simulink model "load_arduino_v_15_loop"  (R2020b)
settings: Solver=FixedStepDiscrete  StartTime=0.0  StopTime=Inf  FixedStep=0.02  RelTol=1e-3  EnableMultiTasking=on
values from neighbouring files (symbols this model uses):
  attuatore_Amax = deg2rad(20)    [AVVIO_YAK_DATA.m]
  attuatore_Amin = deg2rad(-20)    [AVVIO_YAK_DATA.m]
  attuatore_Emax = deg2rad(25)    [AVVIO_YAK_DATA.m]
  attuatore_Emin = deg2rad(-25)    [AVVIO_YAK_DATA.m]
  attuatore_Rmax = deg2rad(25)    [AVVIO_YAK_DATA.m]
  attuatore_Rmin = deg2rad(-25)    [AVVIO_YAK_DATA.m]
  attuatore_Tmax = 0.4    [AVVIO_YAK_DATA.m]
  attuatore_Tmin = 0    [AVVIO_YAK_DATA.m]
  interventoA_05 = 6    [AVVIO_YAK_DATA.m]
  interventoA_1 = 2    [AVVIO_YAK_DATA.m]
  interventoE_05 = 7.5    [AVVIO_YAK_DATA.m]
  interventoE_1 = 3.2    [AVVIO_YAK_DATA.m]
  interventoT = 0.1    [AVVIO_YAK_DATA.m]
  inv_A = 1    [AVVIO_YAK_DATA.m]
  inv_comp_h = 1    [AVVIO_YAK_DATA.m]
  inv_E = 1    [AVVIO_YAK_DATA.m]
  inv_R = 1    [AVVIO_YAK_DATA.m]
  inv_T = 1    [AVVIO_YAK_DATA.m]
  K_AW_B_AP_quota = 1000    [AVVIO_YAK_DATA.m]
  K_AW_B_becc = -250    [AVVIO_YAK_DATA.m]
  K_AW_B_imb = 0    [AVVIO_YAK_DATA.m]
  K_AW_B_roll = 500    [AVVIO_YAK_DATA.m]
  K_imb_inv = -1    [AVVIO_YAK_DATA.m]
  Kd_h_app = 0.085    [AVVIO_YAK_DATA.m]
  Kd_h_flare = 0.01    [AVVIO_YAK_DATA.m]
  Ki_AP_quota_select = 0.014    [AVVIO_YAK_DATA.m]
  Ki_AP_rotta = 0.03    [AVVIO_YAK_DATA.m]
  Ki_AP_vel = 0.001    [AVVIO_YAK_DATA.m]
  Ki_becch = -0.064065    [AVVIO_YAK_DATA.m]
  Ki_h_app = 0.055    [AVVIO_YAK_DATA.m]
  Ki_h_cruise = 0.008    [AVVIO_YAK_DATA.m]
  Ki_h_flare = 0.07    [AVVIO_YAK_DATA.m]
  Ki_roll = 0.025    [AVVIO_YAK_DATA.m]
  Kp_AP_quota_hold_h = 0.15    [AVVIO_YAK_DATA.m]
  Kp_AP_quota_hold_l = 0.7    [AVVIO_YAK_DATA.m]
  Kp_AP_quota_select = 0.014    [AVVIO_YAK_DATA.m]
  Kp_AP_rotta = 0.7    [AVVIO_YAK_DATA.m]
  Kp_AP_vel = 0.02692    [AVVIO_YAK_DATA.m]
  Kp_becch = -0.1918    [AVVIO_YAK_DATA.m]
  Kp_comp_h = 0.035    [AVVIO_YAK_DATA.m]
  Kp_h_app_max = 0.086    [AVVIO_YAK_DATA.m]
  Kp_h_app_min = 0.01    [AVVIO_YAK_DATA.m]
  Kp_h_cruise = 0.04    [AVVIO_YAK_DATA.m]
  Kp_h_flare = 0.1    [AVVIO_YAK_DATA.m]
  Kp_imb = -0.04    [AVVIO_YAK_DATA.m]
  Kp_p = 0.025    [AVVIO_YAK_DATA.m]
  Kp_q = -0.025    [AVVIO_YAK_DATA.m]
  Kp_roll = 0.11    [AVVIO_YAK_DATA.m]
  Kp_Rotta_ATO = 4    [AVVIO_YAK_DATA.m]
  safe_phi = 55    [AVVIO_YAK_DATA.m]
  safe_V = 40    [AVVIO_YAK_DATA.m]
  t_AP = 0.02    [AVVIO_YAK_DATA.m]
  time_alarm_SAFE = 1    [AVVIO_YAK_DATA.m]
  V_max = 35    [AVVIO_YAK_DATA.m]
  V_stall = 15    [AVVIO_YAK_DATA.m]
  vel_wp1_al = 25    [AVVIO_YAK_DATA.m]
  vel_wp2_al = 20    [AVVIO_YAK_DATA.m]
undefined symbols (not defined in the file or in its folder): DiscIntNeverNeededParam, Newton, phi_max, phi_min, Raphson, theta_max, theta_min, tsamp
libraries: simulink_extras x43, arduinolib x26, pid_lib x8, svdutilitieslib x6, simulink x3, dspsigops x3, aerolibtransform2sys x2, aerolibtransform2 x2, cstblocks x1
(part 6 of 8)

== matlab function load_arduino_v_15_loop/AUTOPILOTA/Subsystem1/Subsystem1/APPROACH/MATLAB Function ==
  data: reset input; gamma input; x_f_out output; h_f_out output; xg0 input; k_x_out output; h_c_out output; no_solution output
function [x_f_out,h_f_out,k_x_out,h_c_out,no_solution] = fcn(reset,gamma,xg0)

 

x_f=-200;
h_f=1.5;
%x_f=-300;
%h_f=10;
k_x=0.01;
h_c=-2;
x_td=5;
h_td_dot=-0.1;
x_td_dot=18;
no_solution = 0;

% x_f=-200;
% h_f=5;
% %x_f=-300;
% %h_f=10;
% k_x=0.01;
% h_c=-1;
% x_td=50;
% h_td_dot=-0.15;
% x_td_dot=18;
% no_solution = 0;

% F = [f(x_f,h_f,gamma,xg0); g(h_c,h_f,k_x,gamma); r(h_c,h_f,k_x,x_f,x_td); s(h_c,h_f,k_x,x_f,x_td,h_td_dot,x_td_dot)];
% 
% J = [ df1() df2(gamma) df3() df4();
%       dg1(k_x) dg2() dg3(h_f,h_c) dg4(k_x);
%       dr1(k_x,x_td,x_f) dr2(k_x,x_td,x_f) dr3(k_x,x_td,x_f,h_f,h_c) dr4();
%       ds1(k_x,x_td,x_f,x_td_dot) ds2(k_x,x_td,x_f,x_td_dot,h_f,h_c) ds3(k_x,x_td,x_f,x_td_dot,h_f,h_c) ds4(k_x,x_td,x_f,x_td_dot)]

persistent x x_new cycle_count eps

if (isempty(x) ||  reset == 0)
x = [h_f; x_f; k_x; h_c];
end

if (isempty(x_new) || reset == 0)
x_new = zeros(4,1);
end

if (isempty(eps) || reset == 0)
eps = ones(1,4);
end
   
if (isempty(cycle_count) || reset == 0)
cycle_count = 0;
end




while ~ (eps(1) < 0.1 && eps(2) < 0.1 && eps(3) < 0.1 && eps(4) < 0.1 )

F = [f(x(2),x(1),gamma,xg0); g(x(4),x(1),x(3),gamma); r(x(4),x(1),x(3),x(2),x_td); s(x(4),x(1),x(3),x(2),x_td,h_td_dot,x_td_dot)];

J = [ df1() df2(gamma) df3() df4();
      dg1(x(3)) dg2() dg3(x(1),x(4)) dg4(x(3));
      dr1(x(3),x_td,x(2)) dr2(x(3),x_td,x(2),x(1),x(4)) dr3(x(3),x_td,x(2),x(1),x(4)) dr4();
      ds1(x(3),x_td,x(2),x_td_dot) ds2(x(3),x_td,x(2),x_td_dot,x(1),x(4)) ds3(x(3),x_td,x(2),x_td_dot,x(1),x(4)) ds4(x(3),x_td,x(2),x_td_dot)] ; 
  
  
x_new = x - J^(-1)*F;

eps(1) = abs(x_new(1)-x(1));
eps(2) = abs(x_new(2)-x(2));
eps(3) = abs(x_new(3)-x(3));
eps(4) = abs(x_new(4)-x(4));


x = x_new;

cycle_count = cycle_count + 1;

if cycle_count > 10
   no_solution = 1; 
   break; 
end

end

if (eps(1) < 0.1 && eps(2) < 0.1 && eps(3) < 0.1 && eps(4) < 0.1 )
   
h_f_out = x(1);
x_f_out = x(2);
k_x_out = x(3);
h_c_out = x(4);

else
    
h_f_out = 0;
x_f_out = 0;
k_x_out = 0;
h_c_out = 0;    
end

function y = f(x_f,h_f,gamma,xg0)                 %inizio equazioni sistema non lineare
y = h_f+(x_f-xg0)*tan(gamma);
end

function y = g(h_c,h_f,k_x,gamma)
y = (h_f-h_c)*k_x-tan(gamma);
end

function y = r(h_c,h_f,k_x,x_f,x_td)
y = h_c + (h_f-h_c)*exp(-k_x*(x_td-x_f));
end

function y = s(h_c,h_f,k_x,x_f,x_td,h_td_dot,x_td_dot)
y = h_td_dot + (h_f-h_c)*k_x*x_td_dot*exp(-k_x*(x_td-x_f));        
end                                                                   % fine equazioni sistema non lineare

function y = df1()                                                    %inizio derivate
y = 1;
end

function y = df2(gamma)
y = tan(gamma);
end

function y = df3()
y = 0;
end

function y = df4()
y = 0;
end

function y = dg1(k_x)
y = k_x;
end

function y = dg2()
y = 0;
end

function y = dg3(h_f,h_c)
y = h_f-h_c;
end

function y = dg4(k_x)
y = -k_x;
end

function y = dr1(k_x,x_td,x_f)
y = exp(-k_x*(x_td-x_f));
end

function y = dr2(k_x,x_td,x_f,h_f,h_c)
y = (h_f-h_c)*k_x*exp(-k_x*(x_td-x_f));
end

function y = dr3(k_x,x_td,x_f,h_f,h_c)
y = (h_f-h_c)*(x_f-x_td)*exp(-k_x*(x_td-x_f));
end

function y = dr4()
y = 1;
end

function y = ds1(k_x,x_td,x_f,x_td_dot)
y = k_x*x_td_dot*exp(-k_x*(x_td-x_f));
end

function y = ds2(k_x,x_td,x_f,x_td_dot,h_f,h_c)
y = (h_f-h_c)*k_x^2*x_td_dot*exp(-k_x*(x_td-x_f));
end

function y = ds3(k_x,x_td,x_f,x_td_dot,h_f,h_c)
y = (h_f-h_c)*x_td_dot*exp(-k_x*(x_td-x_f))+(h_f-h_c)*k_x*x_td_dot*(x_f-x_td)*exp(-k_x*(x_td-x_f));
end

function y = ds4(k_x,x_td,x_f,x_td_dot)
y = -k_x*x_td_dot*exp(-k_x*(x_td-x_f));
end



end

== matlab function load_arduino_v_15_loop/Misure Sensori/BMP_280/MATLAB Function ==
  data: rate_l_up output; Cal_alt input; P input; P_int input; P_refer output; P_cal input; rate_l_dw output
function [rate_l_up, P_refer, rate_l_dw]  = fcn( Cal_alt, P,P_int,P_cal)
%#codegen

persistent P_ref rl_up rl_dw

if isempty(P_ref)
    
    P_ref = 101325;
    
end

if isempty(rl_up)
    
    rl_up = 300;
    
end

if isempty(rl_dw)
    
    rl_dw = -300;
    
end

if Cal_alt == 1
    
    P_ref = P;
 
end

if P_int == 1
   
   P_ref = P_cal; 
   rl_up = 20;
   rl_dw = -20;
    
end
    


P_refer = P_ref;

rate_l_up = rl_up;
rate_l_dw = rl_dw;

== matlab function load_arduino_v_15_loop/Misure Sensori/GPS_Venus/Subsystem2/Create_message ==
  data: status output; byte_pack input; messaggio output
function [status,messaggio]  = LETTURA_NMEA(byte_pack)

persistent message counter start_found end_found

status = false;       %ho aggiunto questo
messaggio = uint8(zeros(1,80)) ;
pos_end = uint8(0) ;
M = uint8(length(byte_pack)) ;


if isempty(end_found) 
    end_found = false ;
end 
if isempty(start_found) 
     start_found = false ;
end 
if isempty (counter) 
    counter = uint8(0) ;
end 
if isempty(message)
     message = uint8(zeros(1,80)) ;
end



if start_found == 0 
    for i = uint8(1) : M  
        if byte_pack(i) == '$' 
            message(1:M - (i-1)) = byte_pack(i:end) ;
            counter = M - (i-1) ; 
            start_found = true ;
            break
        end
    end
    
    
elseif start_found == 1
    for i = uint8(1) : M  
        if byte_pack(i) == 13 
            end_found = true ;
            pos_end = i ;
            break
        end
    end
    
    if end_found == 1
        message(counter + 1 : counter + pos_end) = byte_pack(1:pos_end) ;
        status = true;       %ho aggiunto questo
        messaggio = message ;
        end_found = false ;
        counter = M - pos_end ;
        if pos_end == M 
            start_found = false ; 
            message = uint8(zeros(1,80)) ;
        else  
            start_found = true ;
            message(1:(M - pos_end)) = byte_pack(pos_end + 1 : end) ;
            message(M - pos_end +1 : 80) = ...
                uint8(zeros(1,80 - (M - pos_end) )) ;
        end
         

    else 
    message(counter + 1 : M + counter ) = byte_pack ;
    counter = M + counter  ;
   
    end
    
    
 
        
    
    
end

== matlab function load_arduino_v_15_loop/Misure Sensori/GPS_Venus/Subsystem2/Subsystem/MATLAB Function ==
  data: messaggio input; Lat output; Long output; V output; Magnetic_declination output; heading output; fix_mode output; n_sat output; h_mean_sea output; h_WGS84 output; out_prec input; indice_dimario output
function [Lat,Long,V,Magnetic_declination,heading,fix_mode,n_sat,h_mean_sea,h_WGS84,indice_dimario] = parser_NMEA(messaggio,out_prec)
    

messaggio = char(messaggio) ;

comma_gga = uint8(zeros(1,14));
comma_rmc = uint8(zeros(1,12));
star = uint8(0);
dollar = uint8(0);
find_dollar = uint8(0);
find_comma = uint8(0);
message_type = uint8(zeros(1,5));
indice_dimario = uint8(0);





for i=1:length(messaggio)
   if messaggio(i) == '$'
       find_dollar = find_dollar + uint8(1);
   end
   if messaggio(i) == ','
       find_comma = find_comma + uint8(1);
   end
end
    
if (find_dollar == 1 && (find_comma == 12 || find_comma == 14))               % controllo se il numero di $ e , sono corretti all'interno di messaggio
                                                                             % altrimenti il messaggio è corrotto ed in output mando i messaggi
                                                                             % precedenti
dollar= find(messaggio == '$',1);

mess_type = messaggio(dollar(1) + 1 : dollar(1) + 5);                              % è il nome del messaggio arrivato

% decodifica mesaggio RMC

if mess_type == 'GPRMC'
comma_rmc = find(messaggio == ',');                                              % restituisce le posizioni delle virgole all'interno del messaggio
star = find(messaggio == '*');                                               % restituisce la posizione dell'asterisco all'interno del messaggio
dollar = find(messaggio == '$');                                             % restituisce la posizione del dollaro all'interno del messaggio

Lat_1 = str2double(messaggio(comma_rmc(3) + 1 : comma_rmc(3) + 2));
Lat_2 = str2double(messaggio(comma_rmc(3) + 3 : comma_rmc(4) - 1))/60;
Lat = Lat_1 + Lat_2;
if messaggio(comma_rmc(4) + 1) == 'S'
Lat = -Lat; 
end

Long_1 = str2double(messaggio(comma_rmc(5) + 1 : comma_rmc(5) + 3));
Long_2 = str2double(messaggio(comma_rmc(5) + 4 : comma_rmc(6) - 1))/60;
Long = Long_1 + Long_2;
if messaggio(comma_rmc(6) + 1) == 'W'
Long = -Long; 
end

V = str2double(messaggio(comma_rmc(7) + 1 : comma_rmc(8) - 1)); 
    
heading = str2double(messaggio(comma_rmc(8) + 1 : comma_rmc(9) - 1));

Magnetic_declination = str2double(messaggio(comma_rmc(10) + 1 : comma_rmc(11) - 1));
if messaggio(comma_rmc(11) + 1) == 'W'
Magnetic_declination = -Magnetic_declination; 
end

% questi dati non sono presenti nel messaggio rmc, quindi prendo quelli
% precedenti

fix_mode = complex(out_prec(6),0);

n_sat = complex(out_prec(7),0) ;

h_mean_sea = complex(out_prec(8),0) ;

h_WGS84 = complex(out_prec(9),0) ;


%%%%%%%%%%%%%%%%%%%%%%%%%%%%%%%%%%%%%%%%%%%%%%%%%%%%%%%%%

% calcolo checksum

ck_ric = char(zeros(1,2)) ;
ck_ric(1) = messaggio(star(1) + uint8(1))  ;
ck_ric(2) = messaggio(star(1) + uint8(2)) ;

NMEA_rmc_string = uint8(messaggio(dollar(1)+1:star(1)-1)) ;

checksum = uint8(0) ;
for i = 1:length(NMEA_rmc_string) 
    checksum = bitxor(checksum,NMEA_rmc_string(i),'uint8') ;
end

if checksum ~= hex2dec(ck_ric) 
    Lat = out_prec(1) ;
    Long = out_prec(2) ;
    V = out_prec(3) ;
    Magnetic_declination = out_prec(4);
    heading = out_prec(5) ; 
    fix_mode = complex(out_prec(6),0);
    n_sat = complex(out_prec(7),0) ;
    h_mean_sea = complex(out_prec(8),0) ;
    h_WGS84 = complex(out_prec(9),0) ;
    indice_dimario = uint8(10);
end

%%%%%%%%%%%%%%%%%%%%%%%%%%%%%%%%%%%%%%%%%%%%%%%%%%%%%%%%%%%

% decodifica mesaggio GGA

elseif mess_type == 'GPGGA'
comma_gga = find(messaggio == ','); 
star = find(messaggio == '*');
dollar = find(messaggio == '$');


Lat_1 = str2double(messaggio(comma_gga(2) + 1 : comma_gga(2) + 2));
Lat_2 = str2double(messaggio(comma_gga(2) + 3 : comma_gga(3) - 1))/60;
Lat = Lat_1 + Lat_2;
if messaggio(comma_gga(3) + 1) == 'S'
Lat = -Lat; 
end


Long_1 = str2double(messaggio(comma_gga(4) + 1 : comma_gga(4) + 3));
Long_2 = str2double(messaggio(comma_gga(4) + 4 : comma_gga(5) - 1))/60;
Long = Long_1 + Long_2;
if messaggio(comma_gga(5) + 1) == 'W'
Long = -Long; 
end


fix_mode = str2double(messaggio(comma_gga(6) + 1)); 

n_sat = str2double(messaggio(comma_gga(7) + 1 : comma_gga(8) - 1));

h_mean_sea = str2double(messaggio(comma_gga(9) + 1 : comma_gga(10) - 1));

h_WGS84 = str2double(messaggio(comma_gga(11) + 1 : comma_gga(12) - 1));

% questi dati non sono presenti nel messaggio rmc, quindi prendo quelli
% precedenti

V = out_prec(3) ;

Magnetic_declination = out_prec(4);

heading = out_prec(5) ; 

%%%%%%%%%%%%%%%%%%%%%%%%%%%%%%%%%%%%%%%%%%%%%%%%%%%%%%%%%%%%%%%%%%%

% calcolo del checksum
ck_ric = char(zeros(1,2)) ;
ck_ric(1) = messaggio(star(1) + uint8(1))  ;
ck_ric(2) = messaggio(star(1) + uint8(2)) ;

NMEA_gga_string = uint8(messaggio(dollar(1)+1:star(1)-1)) ;

checksum = uint8(0) ;
for i = 1:length(NMEA_gga_string) 
    checksum = bitxor(checksum,NMEA_gga_string(i),'uint8') ;
end

if checksum ~= hex2dec(ck_ric) 
    Lat = out_prec(1) ;
    Long = out_prec(2) ;
    V = out_prec(3) ;
    Magnetic_declination = out_prec(4);
    heading = out_prec(5) ; 
fix_mode = complex(out_prec(6),0);

n_sat = complex(out_prec(7),0) ;

h_mean_sea = complex(out_prec(8),0) ;

h_WGS84 = complex(out_prec(9),0) ;
indice_dimario = uint8(20);
   
    
end

%%%%%%%%%%%%%%%%%%%%%%%%%%%%%%%%%%%%%%%%%%%%%%%%%%%%%%%%%%%%%%%%%%%%
        
else
    
    Lat = out_prec(1) ;
    Long = out_prec(2) ;
    V = out_prec(3) ;
    Magnetic_declination = out_prec(4);
    heading = out_prec(5) ; 
fix_mode = complex(out_prec(6),0);

n_sat = complex(out_prec(7),0) ;

h_mean_sea = complex(out_prec(8),0) ;

h_WGS84 = complex(out_prec(9),0) ; 
   
    
    
end


else
    
    Lat = out_prec(1) ;
    Long = out_prec(2) ;
    V = out_prec(3) ;
    Magnetic_declination = out_prec(4);
    heading = out_prec(5) ; 
    fix_mode = complex(out_prec(6),0);
    n_sat = complex(out_prec(7),0) ;
    h_mean_sea = complex(out_prec(8),0) ;
    h_WGS84 = complex(out_prec(9),0) ; 
end

end

== matlab function load_arduino_v_15_loop/AUTOPILOTA/Subsystem1/Subsystem1/CALIBRATING_HOME_COORDINATES ==
  data: Cal_home input; Lat_Home output; Long_Home output; Lat input; Long input; h input; psi input; h_Home output; psi_Home output; GC_info input; WP_AL input; WP_db_info input
function [Lat_Home,Long_Home,h_Home,psi_Home] = fcn(Cal_home,Lat,Long,h,psi,GC_info,WP_AL,WP_db_info)
%#codegen

persistent Lat_H;
persistent Long_H;
persistent h_H;
persistent psi_H;
persistent counter;

if isempty( Lat_H)
    Lat_H = 0;
end

if isempty(Long_H)
   Long_H = 0;
end

if isempty(h_H)
    h_H = 0;
end

if isempty(psi_H)
    psi_H = 2.8274;        %162deg      (%2.79-160deg)
end

if isempty(counter)
    counter = 1;
end




% if Cal_home(1)==1
%     
%     Lat_H = Lat;
%     Long_H = Long;
%     h_H = h;
%     psi_H = psi;
%     
% end
% 
% if GC_info == 3
%     counter = 1;
%     for indice=1:size(WP_AL,1)
%         if WP_db_info(indice,5)==1
%             counter=indice;
%         end
%     end
% end
% 
% AL = WP_AL(counter,2);
% LatWP = WP_AL(counter,5);
% LongWP = WP_AL(counter,6);
% 
% LatWP2 = WP_AL(counter+1,5);
% LongWP2 = WP_AL(counter+1,6);    
% 
% dr=pi/180;
% 
% if AL == 1
%     Lat_Home = LatWP*dr;
%     Long_Home = LongWP*dr;
%     h_Home = WP_AL(counter,7);
%     psi_Home = atan2(sin(LongWP2*dr-LongWP*dr)*cos(LatWP2*dr),cos(LatWP*dr)*sin(LatWP2*dr)-sin(LatWP*dr)*cos(LatWP2*dr)*cos(LongWP2*dr-LongWP*dr));
% else
%     Lat_Home=Lat_H;
%     Long_Home=Long_H;
%     h_Home=h_H;
%     psi_Home=psi_H;
% end
dr=pi/180;

LatWP = WP_AL(1,5);
LongWP = WP_AL(1,6);

LatWP2 = WP_AL(2,5);
LongWP2 = WP_AL(2,6); 

Lat_Home = LatWP*dr;
Long_Home = LongWP*dr;
h_Home = WP_AL(1,7);
psi_Home = atan2(sin(LongWP2*dr-LongWP*dr)*cos(LatWP2*dr),cos(LatWP*dr)*sin(LatWP2*dr)-sin(LatWP*dr)*cos(LatWP2*dr)*cos(LongWP2*dr-LongWP*dr));

if psi_Home < 0
    psi_Home = 2*pi - abs(psi_Home);
end

== matlab function load_arduino_v_15_loop/AUTOPILOTA/Subsystem1/Subsystem1/CREAZIONE_WAYPOINT /MATLAB Function ==
  data: lat_end output; long_end output; lat_ini input; long_ini input; heading input; distance input


function [lat_end,long_end] = fcn2(lat_ini,long_ini,heading,distance)


lat_end=zeros(1,3);
long_end=zeros(1,3);

R=6378137 ; %Earth Radius  

for n=1:3
    
lat_end(n) = asin(sin(lat_ini)*cos(distance(n)/R) + cos(lat_ini)*sin(distance(n)/R)*cos(heading));
long_end(n) = long_ini + atan2(sin(heading)*sin(distance(n)/R)*cos(lat_ini), cos(distance(n)/R)-sin(lat_ini)*sin(lat_end(n))); 


end


end

== matlab function load_arduino_v_15_loop/MISURE DA SENSORI FILTRATE/TX & RX Seriale Arduino Raspberry/Subsystem1/MATLAB Function ==
  data: byte_pack input; status output; messaggio output
function [status,messaggio]  = LETTURA_Arduino_mex(byte_pack)

persistent message counter start_found

status = false;                                        %ho aggiunto questo
messaggio = uint8(zeros(1,31)) ;
M = uint8(length(byte_pack)) ;


if isempty(start_found) 
     start_found = false ;
end 
if isempty (counter) 
    counter = uint8(0) ;
end 
if isempty(message)
     message = uint8(zeros(1,31)) ;
end


if start_found == 0 
    for i = 1 : M-1  
        if ( byte_pack(i) == 255 &&  byte_pack(i + 1) == 254 )                  % mi conviene mandare un secondo byte all'inizio cosi non devo cambiare nulla
            message(1:M - (i-1)) = byte_pack(i:end) ;
            counter = M - (i-1) ; 
            start_found = true ;
            break
        end
    end   % lho messo qua
        if counter == M 
            messaggio = message ;
            message = uint8(zeros(1,31)) ;
            status = true ;
            start_found = false ;
            counter = uint8(0) ;
        end
     %end
    
    
elseif start_found == 1 

        message(counter + 1 : end) = byte_pack(1:M - counter) ;
        status = true;       %ho aggiunto questo
        messaggio = message ;
        counter = M - counter ;
        message = uint8(zeros(1,31)) ;
        
            for i = counter : M-1  
        if ( byte_pack(i) == 255 &&  byte_pack(i + 1) == 254 )                  % mi conviene mandare un secondo byte all'inizio cosi non devo cambiare nulla
            message(1:M - (i-1)) = byte_pack(i:end) ;
            counter = M - (i-1) ; 
            start_found = true ;
            break
        else 
            start_found = false ;
            counter = uint8(0);
        end 
            end

end





% function [status,messaggio]  = LETTURA_Rasp_mex(byte_pack)
% 
% persistent message counter start_found
% 
% status = false;                                        %ho aggiunto questo
% messaggio = uint8(zeros(1,30)) ;
% M = uint8(length(byte_pack)) ;
% 
% if isempty(start_found) 
%      start_found = false ;
% end 
% if isempty (counter) 
%     counter = uint8(0) ;
% end 
% if isempty(message)
%      message = uint8(zeros(1,30 )) ;
% end
% 
% 
% if  start_found == 0  
%     for i = 1 : M-1  
%         if ( byte_pack(i) == 255 &&  byte_pack(i + 1) == 254 ) 
%             message(1:M - (i-1)) = byte_pack(i:end) ;
%             counter = M - (i-1) ; 
%             start_found = true ;
%             break
%         end
%         if counter == M 
%             messaggio = message ;
%             message = uint8(zeros(1,30 )) ;
%             status = true ;
%             start_found = false ;
%             counter = uint8(0) ;
%         end
%      end
    
%     
% elseif start_found == 1 
% 
%         message(counter + 1 : end) = byte_pack(1:M - counter) ;
%         status = true;       %ho aggiunto questo
%         messaggio = message ;
%         counter = M - counter ;
%         message = uint8(zeros(1,30 )) ;
%         message (1 : M-counter ) = byte_pack(counter + 1:end) ;
%         counter = M - counter ;
% 
% end

== stateflow chart load_arduino_v_15_loop/AIR TX/Enable /Chart ==
  state sendbyte(bt,n) [function]
  state Inputblock
    entry: i=1;
    Inputblock -> (junction 28)
    (junction 32) -> (junction 28) [order 1] : [ i<Len]
        | {i++;}
    (junction 28) -> (junction 32) : {sendbyte(datain,i);}
    (junction 32) -> (junction 48) [order 2] : {i=1;}
  (default) -> Inputblock
  data: bt function_input uint8; n function_input; datain input uint8; Len input uint16 size=1; i local uint8 =0

== stateflow chart load_arduino_v_15_loop/AUTOPILOTA/Subsystem1/Subsystem1/Chart1 ==
  state Allignment1
    du:
    maneuver_selector=1;
    landing_selector=0;
    trig_approach = 0;
    trig_flare = 0;
    approach_selector = 0;
  state Abort
    du:
    maneuver_selector=1;
    landing_selector=0;
    trig_approach = 0;
    trig_flare = 0;
    approach_selector = 0;
  state Allignment
    du:
    trig_flare = 0;
    approach_selector = 0;
    maneuver_selector=1;
    landing_selector=0;
    trig_approach = 0;
  state Approach
    du:
    trig_flare = 0;
    trig_approach = 1;
    approach_selector = 1;
    landing_selector=1;
    maneuver_selector=2;
  state Flare
    du:
    trig_approach = 0;
    trig_flare = 1;
    approach_selector = 0;
    landing_selector=2;
    maneuver_selector=3;
  (default) -> Allignment1 : {maneuver_selector=1;
      |  landing_selector=0;
      |  trig_approach = 0;
      |  trig_flare = 0;
      |  approach_selector = 1;}
  Approach -> Allignment1 [order 2] : [modo ~= 4]
  Flare -> Allignment1 [order 2] : [modo ~= 4]
  Allignment -> Allignment1 [order 2] : [modo ~= 4]
  Approach -> Abort [order 3] : [landing_abort == 1]
  Allignment -> Approach [order 1] : [(h > 35) && (h < 60) && (dist <= h*(1/tan(3*pi/180))+100) && (dist >= h*(1/tan(4*pi/180))+100) && (counter >1)]
  Allignment1 -> Allignment : [modo == 4]
  Approach -> Flare [order 1] : [ (x_e >= x_f) && ((h <= (h_f + 1.5)) ||( h > (h_f - 1)))]
  Flare -> (junction 67) [order 1] : [TAS < 3]{landing_selector=0;}
  data: h input; dist input; counter input; maneuver_selector output; x_e input; x_f input; h_f input; TAS input; landing_selector output; trig_approach output; modo input; trig_flare output; approach_selector output; landing_abort input

== matlab function load_arduino_v_15_loop/AIR TX/Heartbeat/Alarm set ==
  data: Alarm input; H_mav output; Rx_mode input

%%

function H_mav = Allarm_set(Alarm, Rx_mode)
%#cambia lo stato se c'è un allarme attivo
% Allarm: possibili allarmi proveniente dall'autopilota
% Rx_mode: richiesta da parte della stazione di terra
% H_mav: setto i parametri Base_mode e System_status del Heartbeat


H_mav = uint8(Rx_mode); % setta la modalità con quella ricevuta da terra

% se un allarme si attiva ha la precedenza sulla richiesta della QGC

if Alarm(1) == 1 % ovvero l'aereo è entrato in safe e si pone su traettoria circolare di sicurezza
    
    H_mav(1) = uint8(220); % MAV_MODE_AUTO_ARMED
    H_mav(2) = uint8(5);   % MAV_STATE_CRITICAL
%     H_mav(3) = uint8(128); % MAV_MODE_FLAG_SAFETY_ARMED

end

% se l'allareme di intervento pilota è attivo ha precedenza sull'allarm
% sefe per cui bisogna riscrivere lo stato del pilota

if Alarm(2) == 1 % si è attivato l'allarme dell'intervento pilota 
    
    H_mav(1) = uint8(216); % MAV_MODE_GUIDED_ARMED
    H_mav(2) = uint8(4);   % MAV_STATE_ACTIVE
%     H_mav(3) = uint8(8);   % MAV_MODE_FLAG_GUIDED_ENABLED

end

== matlab function load_arduino_v_15_loop/AIR TX/If_subsystem/iflogic_function ==
  data: H50 input; iflogic output; H10 input
function iflogic = fcn(H50,H10)
%#codegen
% prende in ingeresso i counter che contano il tempo
% e dice quale messaggio bisogna inviare in base alle frequenze scelte in
% Heartbeat:            1Hz
% SCALED_IMU:           20Hz
%attitude:              20Hz
%GLOBAL_POSITION_INT:   1Hz
%SYS_STATUS:            3Hz
%VFR_HUD:               2Hz
%SERVO_OUTPUT_RAW       1Hz
%SCALED_PRESSURE        1Hz

if H50 == 1  || H50==3
    iflogic=uint8(26); % SCALED_IMU 20Hz
elseif H50==2 || H50==4
    iflogic=uint8(30); %attitude 20Hz
elseif  H50==0 && H10==2
    iflogic=uint8(33); %GLOBAL_POSITION_INT 1Hz
elseif  H50==0 && H10==6
    iflogic=uint8(34); %GLOBAL_POSITION_INT_RAW 1Hz
elseif  H50==0 && H10==0
    iflogic=uint8(0); %Heartbeat 1Hz
elseif H50==0 && (H10==1 || H10==5 || H10==9)
    iflogic=uint8(1); %SYS_STATUS 3Hz
elseif H50==0 && (H10==3 || H10==8)
    iflogic=uint8(74); %VFR_HUD 2Hz
elseif H50==0 && (H10==7)
    iflogic=uint8(36); %SERVO_OUTPUT_RAW 1Hz
elseif H50==0 && (H10==4)
    iflogic=uint8(29); %SCALED_PRESSURE 1Hz
else
    iflogic=uint8(255); %non esiste nessun messaggio con questo codice
    
end

== matlab function load_arduino_v_15_loop/AIR TX/Waypoints/MATLAB Function ==
  data: WP_info_in input; WP_param_in input; WP_info output; GC_info input; WP_param output
function [WP_info,WP_param] = fcn(WP_info_in,WP_param_in, GC_info)
%#codegen
WP_info=WP_info_in(1,:); %%per sicurezza
WP_param=WP_param_in(1,:); %%per sicurezza
[m,n]=size(WP_info_in);
if GC_info(1)==2
    if GC_info(2)>=0 && GC_info(2)<m %per poter inviare i MISSION_ITEM
        WP_info=WP_info_in(GC_info(2)+1,:);
        WP_param=WP_param_in(GC_info(2)+1,:);
    end
end
if GC_info(1)==3 && GC_info(2)>=0 && GC_info(2)<200 %per poter inviae i MISSION_REQUEST
    WP_info=WP_info_in(GC_info(2)+1,:);
end

== matlab function load_arduino_v_15_loop/AUTOPILOTA/Subsystem1/Subsystem/VETTORIALE ==
  data: V_vett output double; h_vett output double; rotta_vett output double; RC_vett output double; ingaggio_AP_mem output; modo input; IAS input; ALT input; HDG input; I_RC input; ingaggio_AP input; ROTTA input; VELOCITA input; QUOTA input; RC input; HEADING input; TAS input; h input; RC_default input; ingaggio_AP_pre input uint8; modo_pre input; IAS_pre input uint8; ALT_pre input uint8; HDG_pre input uint8; modo_pre_mem output; IAS_pre_mem output uint8; ALT_pre_mem output uint8; HDG_pre_mem output uint8
function [V_vett, h_vett, rotta_vett, RC_vett, ingaggio_AP_mem, modo_pre_mem, IAS_pre_mem, ALT_pre_mem, HDG_pre_mem] = vettoriale(modo, IAS, ALT, HDG, I_RC, ingaggio_AP ,ROTTA, VELOCITA, QUOTA, RC, HEADING, TAS, h, RC_default, ingaggio_AP_pre,modo_pre, IAS_pre, ALT_pre, HDG_pre)
%#codegen

persistent V_ref ALT_ref HDG_ref

if isempty(V_ref)
    
    V_ref = 0;
    
end

if isempty(ALT_ref)
    
    ALT_ref = 0;
    
end

if isempty(HDG_ref)
    
    HDG_ref = 0;
    
end

if (ingaggio_AP ~= ingaggio_AP_pre || modo ~= modo_pre || IAS ~= IAS_pre)
    
    V_ref = TAS;
    
end

if (ingaggio_AP ~= ingaggio_AP_pre || modo ~= modo_pre || ALT ~= ALT_pre)
    
    ALT_ref = h;
    
end

if (ingaggio_AP ~= ingaggio_AP_pre || modo ~= modo_pre || HDG ~= HDG_pre)
    
    HDG_ref = HEADING;
    
end

if (IAS == 1)
    
    V_vett = VELOCITA;
    
else
    
    V_vett = V_ref;
    
end

if (ALT == 1)
    
    h_vett = QUOTA;
    
else
    
   h_vett = ALT_ref;
    
end

if (HDG == 1)
    
    rotta_vett = ROTTA;
    
else
    
  rotta_vett = HDG_ref;
    
end

RC_vett = 0;

if ((h_vett - h) >= 0) 
    
    if (I_RC == 1)
    
        RC_vett = RC;
    
    else
    
        RC_vett = RC_default;
    
    end
    
elseif ((h_vett - h) < 0 ) 
    
    if (I_RC == 1)
    
        RC_vett = -RC;
    
    else
    
        RC_vett = -RC_default;
    
    end 
    
end
    
ingaggio_AP_mem = uint8(ingaggio_AP);
modo_pre_mem = modo;
IAS_pre_mem  = uint8(IAS);
ALT_pre_mem  = uint8(ALT);
HDG_pre_mem  = uint8(HDG);

== matlab function load_arduino_v_15_loop/Misure Sensori/BMP_280/MATLAB Function1 ==
  data: T_0 input; P_ref input; h_ output; P input
function h_  = fcn( T_0, P_ref,P)
%#codegen

g     = 9.81;    %accelerazione di gravità
R_gas = 287.05;  %costante dei gas perfetti
dTdh  = -0.0065; %gradiente termico verticale in atmosfera standard 

T_0        = T_0+273.15;


    
h_ = ((R_gas/g)*log(P_ref/P)*T_0)/(1-(dTdh*0.5*(R_gas/g)*log(P_ref/P)));

== matlab function load_arduino_v_15_loop/AIR RX/MATLAB Function1 ==
  data: Base_mode input; GC_req input; value_c input; WP_info_in input; WP_param_in input; mem_out input; T_number input; T_ref input; Mav_state input; AP_int output; AP_rif output; H_mav output; SyS_data output; GC_info output; WP_db_out output; WP_db_param output; WP_AL output; Val_out_MAV output; T_0 output; AP_int_mem input; Base_mode_to_SF output; test output
function [AP_int, AP_rif, H_mav, SyS_data, GC_info, WP_db_out, WP_db_param,WP_AL, Val_out_MAV, T_0, Base_mode_to_SF, test] =...
    RXelaborazione(Base_mode, GC_req, value_c, WP_info_in, WP_param_in, mem_out, T_number, T_ref, Mav_state, AP_int_mem)
%#codegen
% PARTE PER LA GESTIONE DELLE RICHIESTE DALLA STAZIONE DI TERRA
% GC_req= richiesta della stazione di terra, vettore 2 componenti
%           GC_req(1)=1 :    inviare i parametri a fronte della ricezione del
%                           SET_Request
%                             se GC_req(2)=255 li invia tutti altrimenti
%                             solo 1
% value_c= valore da aggiornare;
% GC_info= necessario per S-function mavlink di trasmissione dipende dal
%               GC_req ricevuto
% WP_db_info= [WP_item255.count,WP_item255.seq,WP_item255.command,WP_item255.frame,
%               WP_item255.current,WP_info[5]=WP_item255.autocontinue]
% WP_db_param= parametri ultimo wp arrivato
% Val_out_MAV= valori aggiornati in uscita per il mavlink di trasmissione
% 
%  mem_out=[msg.sysid; msg.compid;msg.msgid;msg.len;msg.seq;flag]
%
% PARTE PER LA GESTIONE MANUALE AUTOMATICO
%Base_mode: richiesta da parte della stazione di terra di settare una
%           modalità di volo
%H_mav: setto i parametri Base_mode e System_status del Heartbeat di
%           trasmissione
%
%  VARIABILI NECESSARIE ALL'AUTOPILOTA
%AP_interruttori: interruttore di pilota automatico e manuale e modalità
%            [ manuale automatico HDG IAS ALT RC]
%
%AP_riferimenti: valori delle modalità di volo [HDG IAS ALT RC]

persistent riferimenti   % riferimenti delle modalità di volo
persistent WP_dbP WP_dbI WP_dbP_AL % lista dei parametri dei waypoint
persistent test1

nWPmax = uint16(6); % Numero massimo di WP da memorizzare %[MILONE]

% Inizializzazione

if isempty(riferimenti)
    
    riferimenti = single([0; 0; 0; 0; 0; 0; 0; 0; 20; 100; 2; 101325; 15; 0; 0; 0]) ; %valori di riferimento di ["I_HDG", "I_IAS", "I_ALT", "I_RC", "I_WP", "I_ATO", "I_AL" "V_HDG","V_IAS","V_ALT","V_RC","C_P0","C_T0","H_LAT","H_LONG","H_ALT"};]
    
end

if isempty(WP_dbP) || (GC_req(1) == 3 && GC_req(2) == 250)
    
        WP_dbP = single(zeros(nWPmax,7)); % nWPmax righe e 7 colonne
        WP_dbI = uint16(zeros(nWPmax,6)); % nWPmax righe e 6 colonne
        
        
end
if isempty(WP_dbP_AL) || (GC_req(1) == 3 && GC_req(2) == 250)                % introdotto da Sensolini: consente di inviare contemporaneamente wp di navigazione ed atterraggio
    
        WP_dbP_AL = single(zeros(nWPmax,7)); % nWPmax righe e 7 colonne
              
end

if isempty(test1)
    
    test1 = 0;
    
end


%% Parte di richieste da mavlik relativa al messaggio PARAM_SET

GC_info = [GC_req; mem_out(1)]; % GC_req (vettore di due) sarebbe GC_request nella S-Function ed è usato per la funzione di PARAM_SET; 
                                % mem_out(1) sarebbe nella S-Function mem_out[0]=msg.sysid; cioè chi interroga

if GC_info(1) == 1
    
    if GC_info(2) > 0 && GC_info(2) <= 7
        
        if abs(value_c) > 0 % attiva l'interruttore
            
            riferimenti(GC_info(2)) = single(1);
            
            %NB: se arrivano valori maggiori di 1 sempre 1 da in output perchè
            % gli interruttori possono essere solo di tipo 0/1
            % altrimenti l'autopilota si blocca
            
        elseif value_c == 0 % disattiva l'interruttore
            
            riferimenti(GC_info(2)) = single(0);
            
        end
        
    elseif GC_info(2) > 7 && GC_info(2) < 12
        
        riferimenti(GC_info(2)) = single(value_c);
        
    end
    
end

%% Parte relativa al messaggio COMMAND_LONG per la temperatura di riferimento dell'altimetro

if T_number == 13;
    
        riferimenti(T_number) = T_ref;
        
end

%%

Val_out_MAV = riferimenti; % output riferimenti

%% WP set

if GC_info(1) == 3 && GC_info(2) == 200 % arriva il numero dei waypoint
    
     if WP_info_in(1) > nWPmax  %%%ATTENZIONE!!  %[MILONE]
        WP_info_in(1) = nWPmax; % se nWP>nWPmax mi comporto come se avessi ricevuto solo i primi nWPmax
                                % non è ottimale, infatti QGC deve aspettare il time out, ma funziona
                                % va migliorata con una opportuna segnalazione
     end
     
     WP_dbI(:,1) = WP_info_in(1);
     
end

if GC_info(1) == 3 && GC_info(2) < 200 % è arrivato un waypoint
    
    if WP_param_in(2) == 0
    
    WP_dbP(WP_info_in(2)+1,:)   = single(WP_param_in); % 7Parametri. è arrivato il numero WP_info(2) +1 perchè in C si parte da 0
    WP_dbI(WP_info_in(2)+1,2:7) = WP_info_in(2:7);     % 6informazioni. è arrivato il numero WP_info(2)  +1 perchè in C si parte da 0
    
    else
     WP_dbP_AL(WP_param_in(1)+1,:) = single(WP_param_in);
     WP_dbI(WP_info_in(2)+1,2:7) = WP_info_in(2:7);
     
    end
    
end

WP_db_out   = WP_dbI;

WP_db_param = WP_dbP;
WP_AL = WP_dbP_AL;

%for i=1:WP_info_in(1)
%if WP_dbP(WP_info_in(2)+1,2) == 0
%    WP_db_param = WP_dbP;
%    WP_AL = single(zeros(nWPmax,7));
%else
%    WP_db_param = single(zeros(nWPmax,7));
%    WP_AL = WP_dbP;
%end
%end
%% parte di gestione modalità autopilota

H_mav   = uint8(zeros(2,1)); % inizializzo il vettore di output
AP_mode = uint8([0;0]);      % inizializzo il vettore che gli interrutori manuale e automatico

Base_mode_to_SF = uint8(0);

% setto i parametri necessari per l'hearbeat e per l'autopilota

if Base_mode == uint8(0) && Mav_state == uint8(0) % INIZIO: è la condizione che si verifica quando connetto Arduino a QGC, ovvero l'autopilota è in stato Standby
    
    H_mav(1) = uint8(0);         % MAV_MODE_PREFLIGHT
    H_mav(2) = uint8(3);         % MAV_STATE_STANDBY
%     H_mav(3) = uint8(64);        % MAV_MODE_FLAG_MANUAL_INPUT_ENABLED   %% il MAV_MODE_FLAG è commentato perché non lo utilizziamo dato che inviamo nel messaggio dell'heartbeat il MAV_MODE in corrispondenza del valore di base_mode (vedere la pagina web MAV'RIC)
    AP_mode  = uint8([1; 0]);    % attivo il manuale  spengo l'automatico
    Base_mode_to_SF = uint8(0);

elseif Base_mode == uint8(0) && Mav_state == uint8(3) % è arrivato MAV_MODE_PREFLIGHT e MAV_STATE_STANDBY (modalità Ready)
    
    H_mav(1) = uint8(0);         % MAV_MODE_PREFLIGHT
    H_mav(2) = uint8(3);         % MAV_STATE_STANDBY
%     H_mav(3) = uint8(64);        % MAV_MODE_FLAG_MANUAL_INPUT_ENABLED 
    AP_mode  = uint8([1; 0]);    % attivo il manuale  spengo l'automatico
    Base_mode_to_SF = uint8(0);
    test1 = 0;

elseif Base_mode == uint8(0) && Mav_state == uint8(2) % è arrivato MAV_MODE_PREFLIGHT e MAV_STATE_CALIBRATING
    
    H_mav(1) = uint8(0);         % MAV_MODE_PREFLIGHT
    H_mav(2) = uint8(2);         % MAV_STATE_CALIBRATING
%     H_mav(3) = uint8(64);        % MAV_MODE_FLAG_MANUAL_INPUT_ENABLED
    AP_mode  = uint8([1; 0]);    % attivo il manuale  spengo l'automatico
    Base_mode_to_SF = uint8(0);
    test1 = 0;
    
elseif Base_mode == uint8(0) && Mav_state == uint8(1) % è arrivato MAV_MODE_PREFLIGHT e MAV_STATE_BOOT
    
    H_mav(1) = uint8(0);         % MAV_MODE_PREFLIGHT
    H_mav(2) = uint8(1);         % MAV_STATE_BOOT
%     H_mav(3) = uint8(64);        % MAV_MODE_FLAG_MANUAL_INPUT_ENABLED
    AP_mode  = uint8([0; 1]);    % In questo caso si attiva l'interrutore di modalità automatica. 
                                 % Il motivo è dovuto al fatto che per fare la prova del safe è necessario che sia attivo 
                                 % il modo automatico altrimenti il safe non entra.
    Base_mode_to_SF = uint8(0);
    test1 = 1;
    
% elseif Base_mode==uint8(80)  %è arrivato MAV_MODE_STABILIZE_DISARMED, 1 manual in QGC
%     H_mav(1)=uint8(80);        %MAV_MODE_GUIDED_ARMED
%     H_mav(2)=uint8(4);          %MAV_STATE_ACTIVE
%     AP_mode=uint8([1; 0]);      %attivo il manuale  spengo l'automatico

elseif Base_mode == uint8(192) % è arrivato MAV_MODE_MANUAL_ARMED
    
    H_mav(1) = uint8(192);       % MAV_MODE_MANUAL_ARMED 
    H_mav(2) = uint8(4);         % MAV_STATE_ACTIVE
%     H_mav(3) = uint8(64);        % MAV_MODE_FLAG_MANUAL_INPUT_ENABLED
    AP_mode  = uint8([1; 0]);    % attivo il manuale  spengo l'automatico
    Base_mode_to_SF = uint8(192);
    
elseif Base_mode == uint8(208) % è arrivato MAV_MODE_STABILIZE_ARMED (sarebbe la modalità Stand By presente nello State Flow degli stati)
    
    H_mav(1) = uint8(208);       % MAV_MODE_STABILIZE_ARMED
    H_mav(2) = uint8(3);         % MAV_STATE_STANDBY
%     H_mav(3) = uint8(64);        % MAV_MODE_FLAG_MANUAL_INPUT_ENABLED
    AP_mode  = uint8([0; 0]);    % disattiva l'interruttore del manuale ma l'automatico non è ancora attivo
    Base_mode_to_SF = uint8(208);

elseif Base_mode == uint8(220) && Mav_state ~= uint8(5) % è arrivato MAV_MODE_AUTO_ARMED
    
    if (AP_int_mem(1) == uint8(0) && AP_int_mem(2) == uint8(0) && ((AP_int_mem(3) == uint8(1) || AP_int_mem(4) == uint8(1) ||...
        AP_int_mem(5) == uint8(1) || AP_int_mem(6) == uint8(1) || AP_int_mem(7) == uint8(1) || AP_int_mem(8) == uint8(1))))
    
        H_mav(1) = uint8(220);       % MAV_MODE_AUTO_ARMED
        H_mav(2) = uint8(4);         % MAV_STATE_ACTIVE
%         H_mav(3) = uint8(4);         % MAV_MODE_FLAG_AUTO_ENABLED
        AP_mode  = uint8([0; 1]);    % spengo il manuale attivo l'automatico
        Base_mode_to_SF = uint8(220);
        
    elseif (AP_int_mem(1) == uint8(0) && AP_int_mem(2) == uint8(1) && ((AP_int_mem(3) == uint8(1) || AP_int_mem(4) == uint8(1) ||...
            AP_int_mem(5) == uint8(1) || AP_int_mem(6) == uint8(1) || AP_int_mem(7) == uint8(1) || AP_int_mem(8) == uint8(1)))) 
        
        H_mav(1) = uint8(220);       % MAV_MODE_AUTO_ARMED
        H_mav(2) = uint8(4);         % MAV_STATE_ACTIVE
        AP_mode  = uint8([0; 1]);    % spengo il manuale attivo l'automatico
        Base_mode_to_SF = uint8(220);
        
    else 
        
        H_mav(1)  = uint8(208);       % MAV_MODE_STABILIZE_ARMED
        H_mav(2)  = uint8(3);         % MAV_STATE_STANDBY
        AP_mode   = uint8([0; 0]);    % attivo il manuale  spengo l'automatico
        Base_mode_to_SF = uint8(208);
    
    end

% elseif Base_mode == uint8(216)  % è arrivato MAV_MODE_GUIDED_ARMED
%     
%     H_mav(1) = uint8(8);         % MAV_MODE_FLAG_GUIDED_ENABLED
%     H_mav(2) = uint8(4);         % MAV_STATE_ACTIVE
%     AP_mode  = uint8([0; 1]);    % spengo il manuale attivo l'automatico
    
elseif Mav_state == uint8(5)  % si verifica nell'S-Function di ricezione quando il velivolo è andato in safe ovvero quando Alarm_Safe = 1
    
    H_mav(1) = uint8(220);      % MAV_MODE_AUTO_ARMED
    H_mav(2) = uint8(5);        % MAV_STATE_CRITICAL
%     H_mav(3) = uint8(128);      % MAV_MODE_FLAG_SAFETY_ARMED
    AP_mode  = uint8([0; 1]);   % spengo il manuale attivo l'automatico

% elseif Base_mode==uint8(66) % è arrivato MAV_MODE_TEST_DISARMED, lo usiamo per fare la calibrazione
%     H_mav(1)=uint8(64);        %MAV_MODE_FLAG_MANUAL_INPUT_ENABLED
%     H_mav(2)=uint8(2);         %MAV_STATE_CALIBRATING
%     AP_mode=uint8([1; 0]);     %attivo il manuale  spengo l'automatico
    
    %%%%%%%%%%%%%%%%%%%%%%%%%%%
    % elseif Base_mode==uint8(192) %%ARMED PREFLIGHT
    %     H_mav(1)=uint8(192);        %MAV_MODE_FLAG_MANUAL_INPUT_ENABLED
    %     H_mav(2)=uint8(3);          %	MAV_STATE_EMERGENCY
    %     AP_mode=uint8([0; 1]);     %spengo il manuale attivo l'automatico
    %     elseif Base_mode==uint8(64) %%DISARMED PREFLIGHT
    %     H_mav(1)=uint8(64);        %MAV_MODE_FLAG_MANUAL_INPUT_ENABLED
    %     H_mav(2)=uint8(3);          %	MAV_STATE_EMERGENCY
    %     AP_mode=uint8([0; 1]);     %spengo il manuale attivo l'automatico
    %     %%%%%%%%%%%%%%%%%%%%%%%%%%%%%%%%%%%%%%%

else
    
    H_mav(1) = uint8(192);       % MAV_MODE_MANUAL_ARMED 
    H_mav(2) = uint8(6);         % MAV_STATE_EMERGENCY
%     H_mav(3) = uint8(64);        % MAV_MODE_FLAG_MANUAL_INPUT_ENABLED
    AP_mode  = uint8([1; 0]);    % attivo il manuale  spengo l'automatico
    
end

%% parte delle informazioni sullo stato del sistema in ricezione

% calcolo dei messaggi persi provenienti dalla stazione di terra

drop_rate = 10*((100*mem_out(6))/mem_out(5));  % 10*percentuale !non moltipilicare direttamente per 10000 perchè è un uint16 e va in overflow
SyS_data  = [drop_rate mem_out(7) mem_out(3)];

%% parte per settare gli interrutori e i riferimenti

AP_int = [AP_mode; uint8(riferimenti(1:7))]; % interruttori
AP_rif = riferimenti(8:11);                  % riferimenti

T_0 = riferimenti(13); % valore della temperatura di riferimento T_0 dell'altimetro

test = test1;

== matlab function load_arduino_v_15_loop/Misure Sensori/X-Sense MTi/MATLAB Function1 ==
  data: Messaggio input; Mex_out output; Mex_prec input; Control output
function [Mex_out,Control]  = checksum_control(Messaggio,Mex_prec)

Control = uint8(0);

mti_string = uint8(Messaggio(2:41));

checksum = sum(mti_string) ; 

hex_checksum = dec2hex(checksum);

if ((hex_checksum(3) == '0') && (hex_checksum(4) == '0'))
    Mex_out = uint8(Messaggio);

else
   Control = uint8(1); 
   Mex_out = Mex_prec;   
end



end
